simulink model "finaleproject_new_18"  (R2018b)
settings: Solver=VariableStepAuto  StartTime=0.0  StopTime=30  RelTol=1e-3
undefined symbols (not defined in the file): Ion, Lithium, sigbuilder_block
libraries: powerlib x21, simulink x6, electricdrivelib x2, powerlib_meascontrol x1, eePwmGenerator x1, re_lib x1
settings Model: Creator=ACER  LastModifiedBy=ACER
settings SolverCC: ZeroCrossAlgorithm=Adaptive
settings DataIOCC: ReturnWorkspaceOutputs=on
settings DebuggingCC: IgnoredZcDiagnostic=none  UnconnectedInputMsg=none  UnconnectedOutputMsg=none  UnconnectedLineMsg=none  SFMachineParentedDataDiag=error
settings ModelReferenceCC: EnableRefExpFcnMdlSchedulingChecks=off
settings RTWCC: Description=Generic Real-Time Target

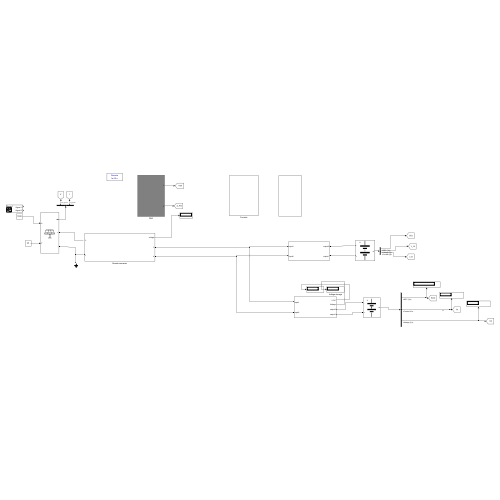
[thumbnail: Simulink's stored preview of the top-level diagram]
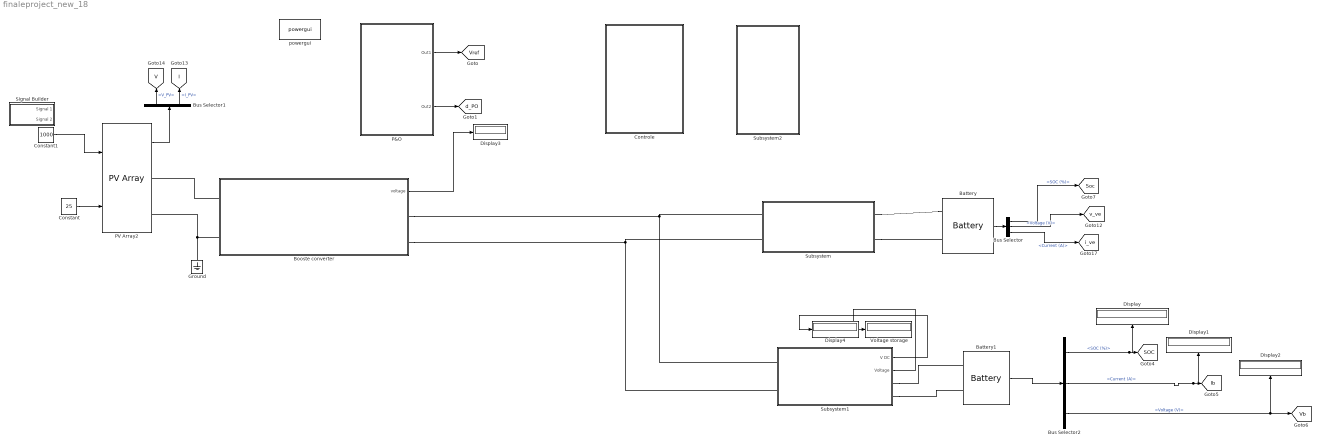
== system finaleproject_new_18 ==
  Battery : electricdrivelib/Extra Sources/Battery  BatType=Lithium-Ion  ShowTempParam=off  ThermalPreset=no  ShowAgeParam=off  NomV=400  NomQ=125  SOC=79.9  Batt_Tr=0.0001  PresetModel=on  MaxQ=125  MinV=300  FullV=465.5949  Dis_rate=54.3478  R=0.032  Normal_OP=113.0435  expZone="[432.1543      6.141304]"  current=[6.5 13 32.5]  Units=Time  Tci=20  NomT=20  T2=-30  MaxQ2=4.8  FullV2=7.1  Normal_OP2=5.655  expZone2="[6.58           1]"  Rca=0.6  ti=2000  Dp=0  Neq0=0  Tsim=1e6  Ta1=25  Qeol=5.4*0.9  Reol=0.013333*1.2  Char_age=[2.3478, 3]  Dis_age=[2.3478, 10]  N1=1500  N2=10500  N3=1000  N4=1400  Ta2=45  N5=950
  Battery1 : electricdrivelib/Extra Sources/Battery  BatType=Lithium-Ion  ShowTempParam=off  ThermalPreset=no  ShowAgeParam=off  NomV=300  NomQ=200*6  SOC=80  Batt_Tr=0.0001  PresetModel=on  MaxQ=1200  MinV=225  FullV=349.1961  Dis_rate=521.7391  R=0.0025  Normal_OP=1085.2174  expZone="[324.1158      58.95652]"  current=[6.5 13 32.5]  Units=Time  Tci=20  NomT=20  T2=-30  MaxQ2=4.8  FullV2=7.1  Normal_OP2=5.655  expZone2="[6.58           1]"  Rca=0.6  ti=2000  Dp=0  Neq0=0  Tsim=1e6  Ta1=25  Qeol=5.4*0.9  Reol=0.013333*1.2  Char_age=[2.3478, 3]  Dis_age=[2.3478, 10]  N1=1500  N2=10500  N3=1000  N4=1400  Ta2=45  N5=950
  Booste converter : Subsystem
  Bus Selector : BusSelector  OutputSignals=SOC (%),Voltage (V),Current (A)
  Bus Selector1 : BusSelector  OutputSignals=V_PV,I_PV
  Bus Selector2 : BusSelector  OutputSignals=SOC (%),Current (A),Voltage (V)
  Constant : Constant  Value=25
  Constant1 : Constant  Value=1000
  Controle : Subsystem
  Display{,1..4} (5 alike) : Display
  Ground : powerlib/Elements/Ground  LConnTagsString=a
  P&O : Subsystem
  PV Array2 : re_lib/Solar/PV Array  Npar=8*6  Nser=10  PlotType=array @ 1000 W/m2 & specified temperatures  S_vec="[ 1000  500  100 ]"  Temp_C_vec="[  25  ]"  ModuleName=User-defined  PlotWhenSelected=off  Pm=210.18  Ncell=72  Voc=45.90  Isc=6  Vm=37.20  Im=5.65  beta_Voc_pc=-0.36099  alpha_Isc_pc=0.102  beta_Voc=-0.16569  alpha_Isc=0.00612  IL=6.0381  I0=2.2435e-10  nI=1.0339  Rsh=465.1473  Rs=0.54298  RobustModel=off  RobustCellTemperature=25  BAL=on  Tc=1e-6  Tfilter=5e-5
  Signal Builder : Subsystem  Tag=STV Subsys  LoadFcn=sigbuilder_block('load');  StartFcn=sigbuilder_block('start');  StopFcn=sigbuilder_block('stop');  ClipboardFcn=sigbuilder_block('clipboard');  mask(Sigbuilder block){tuvar=[0:10]}
      mask help: Simulink:masks:SigbuilderBlock_MD
      mask init:
      | if ~strcmp(get_param(bdroot(gcbh),'SimulationStatus'),'stopped') tuvar = sigbuilder_block('maskInit'); end
      settings: CopyFcn=sigbuilder_block('copy');  DeleteFcn=sigbuilder_block('delete');  ModelCloseFcn=sigbuilder_block('modelClose');  PreSaveFcn=sigbuilder_block('preSave');  PauseFcn=sigbuilder_block('pause');  ContinueFcn=sigbuilder_block('continue');  NameChangeFcn=sigbuilder_block('namechange');  OpenFcn=sigbuilder_block('open',[204.5 106 550.5 362.5 ]);  CloseFcn=sigbuilder_block('close');
      mask Display: plot(0, 0, 100, 100,[2, 2, 32, 32, 2], [68, 8, 8, 68, 68],[32, 2], [38, 38], [32, 19, 2],[53, 60, 44], [32, 17, 17, 2],[16, 16, 31, 31]);txt = getActiveGroup(gcbh);text(2, 100, txt,'verticalAlignment', 'top');
  Subsystem : Subsystem
  Subsystem1 : Subsystem
  Subsystem2 : Subsystem
  Voltage storage : Display
  powergui : powerlib/powergui  Priority=1  SimulationMode=Discrete  SampleTime=10e-6  frequency=60  Iterations=50  frequencyindice=0  Pbase=100e6  ErrMax=1e-4  UnitsV=kV  UnitsW=MW  buscounter=0  FunctionMessages=off  echomessages=off  EnableUseOfTLC=off  CurrentSourceSwitches=off  DisableSnubberDevices=off  DisableRonSwitches=off  DisableVfSwitches=off  DisplayEquations=off  AutomaticDiscreteSolvers=off  SolverType=Tustin/Backward Euler (TBE)  Interpol=off  ExternalGateDelay=off  methode=off  Ts=100  x0status=blocks  SPID=on  SwTol=0  HookPort=off  NonlinearTolerance=1e-4  nMaxIteration=100  ContinueOnMaxIteration=off  RestoreLinks=warning  ResistiveCurrentMeasurement=off  Frange=[0:2:500]  Ylog=off  Xlog=on  ShowGrid=off  save=off  variable=ZData  structure=0  ZoomFFT=off  StartTime=0.0  cycles=1  DisplayStyle=1  fundamental=60  FreqAxis=off  MaxFrequency=1000  frequencyindicesteady=1  RmsSteady=1  display=off
  tag scope: I=global, Ib=global, SOC=global, Soc=global, V=global, Vb=global, Vref=global, d_PO=global, i_ve=global, v_ve=global
  wires:
  Constant1/1 -> PV Array2/1
  Bus Selector2/2 -> [Ib], Display1/1  "<Current (A)>"
  Bus Selector/2 -> [v_ve]  "<Voltage (V)>"
  Battery/1 -> Bus Selector/1
  P&O/2(Out2) -> [d_PO]
  PV Array2/1 -> Bus Selector1/1
  Bus Selector/1 -> [Soc]  "<SOC (%)>"
  Bus Selector/3 -> [i_ve]  "<Current (A)>"
  Bus Selector1/1 -> [V]  "<V_PV>"
  Bus Selector2/3 -> [Vb], Display2/1  "<Voltage (V)>"
  Constant/1 -> PV Array2/2
  Battery1/1 -> Bus Selector2/1
  Booste converter/1(voltage) -> Display3/1
  Bus Selector1/2 -> [I]  "<I_PV>"
  P&O/1(Out1) -> [Vref]
  Bus Selector2/1 -> Display/1, [SOC]  "<SOC (%)>"
  Subsystem1/2(Voltage) -> Voltage storage/1
  Subsystem1/1(V DC) -> Display4/1
  connections:
  Booste converter/LConn2 -- PV Array2/RConn2 -- Ground/LConn1
  Subsystem/RConn1 -- Battery/LConn2
  Subsystem/RConn2 -- Battery/LConn1
  Subsystem1/RConn1 -- Battery1/LConn2
  Booste converter/LConn1 -- PV Array2/RConn1
  Subsystem1/RConn2 -- Battery1/LConn1
  Booste converter/RConn1 -- Subsystem/LConn1 -- Subsystem1/LConn1
  Booste converter/RConn2 -- Subsystem/LConn2 -- Subsystem1/LConn2

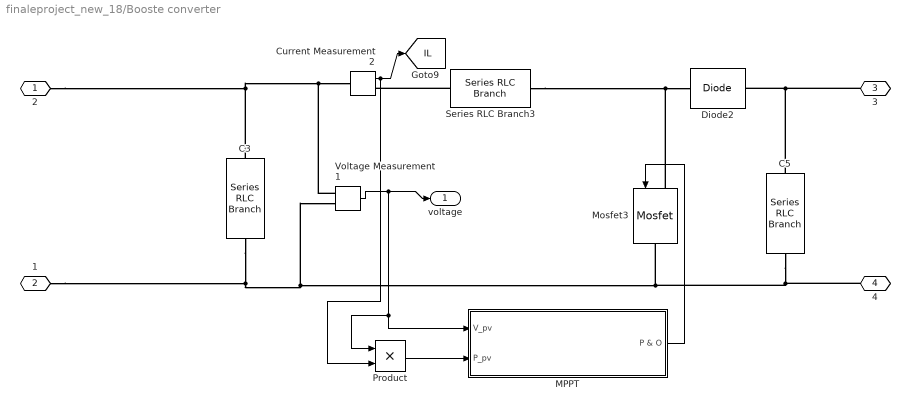
== system finaleproject_new_18/Booste converter ==
  C3 : powerlib/Elements/Series RLC Branch  LConnTagsString=__new0  RConnTagsString=__new0  BranchType=C  Resistance=0.1  Inductance=0.0078  SetiL0=off  InitialCurrent=0  Capacitance=470e-6  Setx0=on  InitialVoltage=400  Measurements=None
  C5 : powerlib/Elements/Series RLC Branch  LConnTagsString=__new0  RConnTagsString=__new0  BranchType=C  Resistance=0.1  Inductance=0.0078  SetiL0=off  InitialCurrent=0  Capacitance=222e-6  Setx0=off  InitialVoltage=500  Measurements=None
  Current Measurement2 : powerlib/Measurements/Current Measurement  PhasorSimulation=off  OutputType=Complex  PSBequivalent=0
  Diode2 : powerlib/Power Electronics/Diode  Ron=0.001  Lon=0  Vf=0.8  IC=0  UseSnubber=off  Rs=500  Cs=250e-9  Measurements=off
  MPPT : Subsystem
  Mosfet3 : powerlib/Power Electronics/Mosfet  Ron=0.1  Lon=0  Rd=0.01  Vfd=0  IC=0  Rs=1e5  Cs=inf  Measurements=off
  Product : Product
  Series RLC Branch3 : powerlib/Elements/Series RLC Branch  LConnTagsString=__new0  RConnTagsString=__new0  BranchType=L  Resistance=0.1  Inductance=2.25e-3  SetiL0=off  InitialCurrent=0  Capacitance=1e-6  Setx0=off  InitialVoltage=0  Measurements=None
  Voltage Measurement1 : powerlib/Measurements/Voltage Measurement  PhasorSimulation=off  OutputType=Complex  PSBequivalent=0
  2 : PMIOPort  Side=Left
  1 : PMIOPort  Port=2  Side=Left
  3 : PMIOPort  Port=3  Side=Right
  4 : PMIOPort  Port=4  Side=Right
  voltage : Outport
  tag scope: IL=global
  wires:
  Current Measurement2/1 -> Product/2, [IL]
  Voltage Measurement1/1 -> Product/1, MPPT/1(V_pv), voltage/1
  Product/1 -> MPPT/2(P_pv)
  MPPT/1(P & O) -> Mosfet3/1
  connections:
  Series RLC Branch3/RConn1 -- Diode2/LConn1 -- Mosfet3/LConn1
  C5/LConn1 -- Diode2/RConn1 -- 3/RConn1
  Voltage Measurement1/LConn1 -- C3/LConn1 -- 2/RConn1 -- Current Measurement2/LConn1
  4/RConn1 -- C5/RConn1 -- Mosfet3/RConn1 -- C3/RConn1 -- 1/RConn1 -- Voltage Measurement1/LConn2
  Series RLC Branch3/LConn1 -- Current Measurement2/RConn1

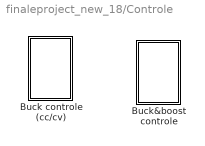
== system finaleproject_new_18/Controle ==
  "Buck controle (cc/cv) " : Subsystem
  Buck&boost controle : Subsystem

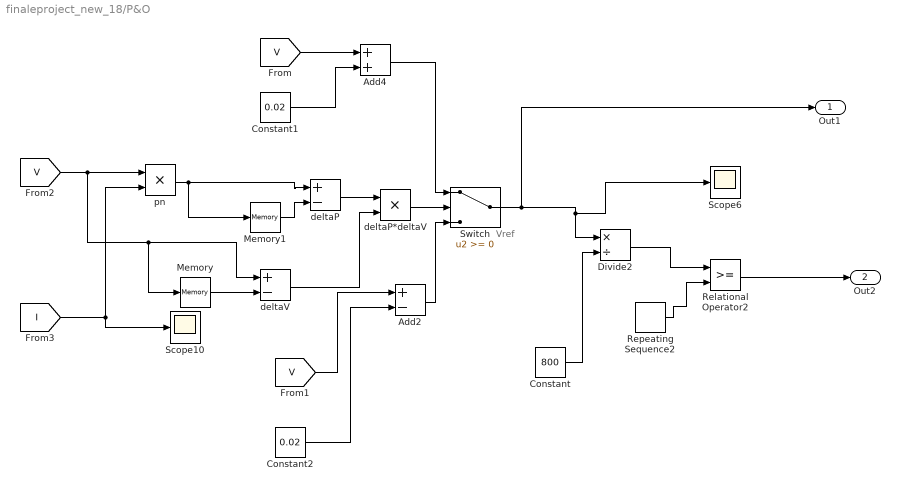
== system finaleproject_new_18/P&O ==
  note: Vref
  Add2 : Sum  Inputs=+-
  Add4 : Sum
  Constant : Constant  Value=800
  Constant1 : Constant  Value=0.02
  Constant2 : Constant  Value=0.02
  Divide2 : Product  Inputs=*/
  Memory : Memory
  Memory1 : Memory
  Relational Operator2 : RelationalOperator  OutDataTypeStr=boolean  RndMeth=Nearest
  Repeating Sequence2 : simulink/Sources/Repeating Sequence  rep_seq_t=[0 1/5000]  rep_seq_y=[0 1]
  Scope10 : Scope
  Scope6 : Scope
  Switch : Switch
  deltaP : Sum  Inputs=+-
  deltaP*deltaV : Product
  deltaV : Sum  Inputs=+-
  pn : Product
  Out1 : Outport  VectorParamsAs1DForOutWhenUnconnected=off
  Out2 : Outport  Port=2  VectorParamsAs1DForOutWhenUnconnected=off
  wires:
  pn/1 -> Memory1/1, deltaP/1
  Constant1/1 -> Add4/2
  Add2/1 -> Switch/3
  deltaP*deltaV/1 -> Switch/2
  [V] -> Add4/1
  Add4/1 -> Switch/1
  deltaP/1 -> deltaP*deltaV/1
  [V] -> deltaV/1, Memory/1, pn/1
  [I] -> pn/2, Scope10/1
  deltaV/1 -> deltaP*deltaV/2
  Memory/1 -> deltaV/2
  Relational Operator2/1 -> Out2/1
  Constant2/1 -> Add2/2
  [V] -> Add2/1
  Repeating Sequence2/1 -> Relational Operator2/2
  Divide2/1 -> Relational Operator2/1
  Memory1/1 -> deltaP/2
  Switch/1 -> Out1/1, Scope6/1, Divide2/1
  Constant/1 -> Divide2/2

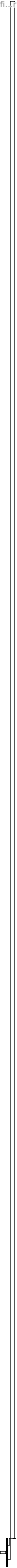
== system finaleproject_new_18/Signal Builder ==
  Demux : Demux  Tag=STV Demux  Outputs=2
      settings: DisplayOption=none
  FromWs : FromWorkspace  Tag=STV FromWs  VariableName=tuvar
      SigBuilderData=|
      | common.afterFinalStr = 'Extrapolate'
      | common.sampleTime = 0
      | dataSet.timeRange = [0 30]
      | dataSet.name = 'Group 1'
      | sbobj.Groups.Name = 'Group 1'
      | sbobj.Groups.Signals(1).Name = 'Signal 1'
      | sbobj.Groups.Signals(1).XData = [0 4 9.85 11 12 12 30]
      | sbobj.Groups.Signals(1).YData = [1000 1005 925 865 760 195 205]
      | sbobj.Groups.Signals(2).Name = 'Signal 2'
      | sbobj.Groups.Signals(2).XData = [0 5 5 30]
      | sbobj.Groups.Signals(2).YData = [0 0 1 1]
      | sbobj.Groups.TimeRange = [0 30]
  Signal 1 : Outport  Tag=STV Outport
  Signal 2 : Outport  Tag=STV Outport  Port=2
  wires:
  Demux/1 -> Signal 1/1
  FromWs/1 -> Demux/1
  Demux/2 -> Signal 2/1

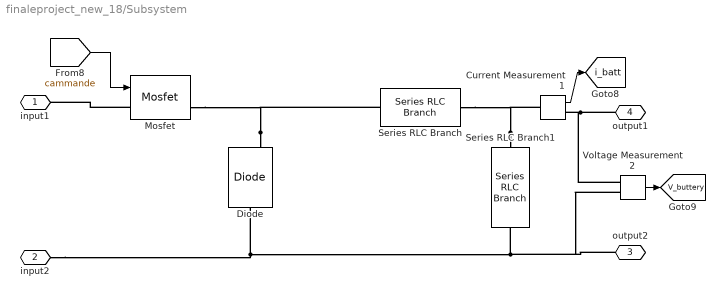
== system finaleproject_new_18/Subsystem ==
  Current Measurement1 : powerlib/Measurements/Current Measurement  PhasorSimulation=off  OutputType=Complex  PSBequivalent=0
  Diode : powerlib/Power Electronics/Diode  Ron=0.001  Lon=0  Vf=0.8  IC=0  UseSnubber=0  Rs=500  Cs=250e-9  Measurements=on
  Mosfet : powerlib/Power Electronics/Mosfet  Ron=0.1  Lon=0  Rd=0.01  Vfd=0  IC=0  Rs=1e5  Cs=inf  Measurements=on
  Series RLC Branch : powerlib/Elements/Series RLC Branch  LConnTagsString=__new0  RConnTagsString=__new0  BranchType=L  Resistance=1  Inductance=2.13e-3  SetiL0=off  InitialCurrent=0  Capacitance=1e-6  Setx0=off  InitialVoltage=0  Measurements=None
  Series RLC Branch1 : powerlib/Elements/Series RLC Branch  LConnTagsString=__new0  RConnTagsString=__new0  BranchType=C  Resistance=1  Inductance=1e-3  SetiL0=off  InitialCurrent=0  Capacitance=47e-6  Setx0=off  InitialVoltage=0  Measurements=None
  Voltage Measurement2 : powerlib/Measurements/Voltage Measurement  PhasorSimulation=off  OutputType=Complex  PSBequivalent=0
  input1 : PMIOPort  Side=Left
  input2 : PMIOPort  Port=2  Side=Left
  output2 : PMIOPort  Port=3  Side=Right
  output1 : PMIOPort  Port=4  Side=Right
  tag scope: V_buttery=global, i_batt=global
  wires:
  Current Measurement1/1 -> [i_batt]
  [cammande] -> Mosfet/1
  Voltage Measurement2/1 -> [V_buttery]
  connections:
  Voltage Measurement2/LConn1 -- output1/RConn1 -- Current Measurement1/RConn1
  Series RLC Branch1/LConn1 -- Series RLC Branch/RConn1 -- Current Measurement1/LConn1
  Diode/RConn1 -- Mosfet/RConn1 -- Series RLC Branch/LConn1
  input2/RConn1 -- Diode/LConn1 -- Voltage Measurement2/LConn2 -- output2/RConn1 -- Series RLC Branch1/RConn1
  Mosfet/LConn1 -- input1/RConn1

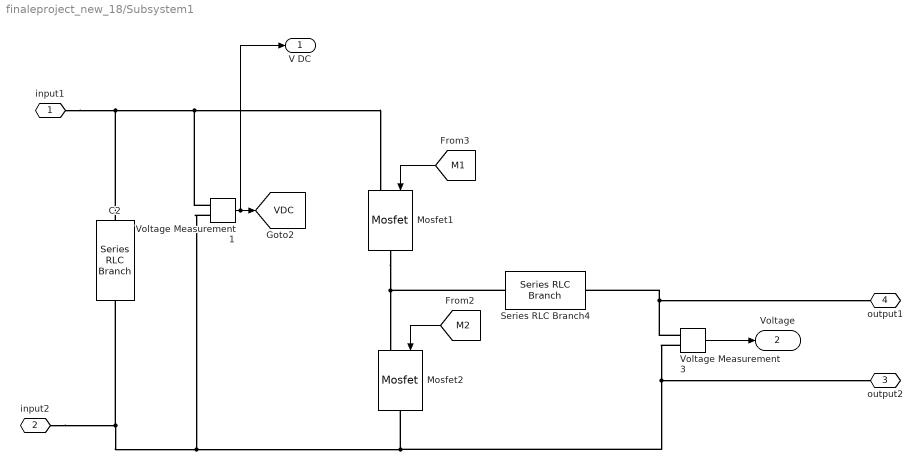
== system finaleproject_new_18/Subsystem1 ==
  C2 : powerlib/Elements/Series RLC Branch  LConnTagsString=__new0  RConnTagsString=__new0  BranchType=C  Resistance=0.01  Inductance=0.0078  SetiL0=off  InitialCurrent=0  Capacitance=5000e-6  Setx0=off  InitialVoltage=0  Measurements=None
  Mosfet1 : powerlib/Power Electronics/Mosfet  Ron=0.1  Lon=0  Rd=0.01  Vfd=0  IC=0  Rs=1e5  Cs=inf  Measurements=off
  Mosfet2 : powerlib/Power Electronics/Mosfet  Ron=0.1  Lon=0  Rd=0.01  Vfd=0  IC=0  Rs=1e5  Cs=inf  Measurements=off
  Series RLC Branch4 : powerlib/Elements/Series RLC Branch  LConnTagsString=__new0  RConnTagsString=__new0  BranchType=L  Resistance=0.05  Inductance=2.2e-3  SetiL0=off  InitialCurrent=0  Capacitance=1e-6  Setx0=off  InitialVoltage=0  Measurements=None
  Voltage Measurement1 : powerlib/Measurements/Voltage Measurement  PhasorSimulation=off  OutputType=Complex  PSBequivalent=0
  Voltage Measurement3 : powerlib/Measurements/Voltage Measurement  PhasorSimulation=off  OutputType=Complex  PSBequivalent=0
  input1 : PMIOPort  Side=Left
  input2 : PMIOPort  Port=2  Side=Left
  output2 : PMIOPort  Port=3  Side=Right
  output1 : PMIOPort  Port=4  Side=Right
  V DC : Outport
  Voltage : Outport  Port=2
  tag scope: VDC=global
  wires:
  Voltage Measurement3/1 -> Voltage/1
  [M1] -> Mosfet1/1
  [M2] -> Mosfet2/1
  Voltage Measurement1/1 -> V DC/1, [VDC]
  connections:
  input2/RConn1 -- Voltage Measurement1/LConn2 -- Voltage Measurement3/LConn2 -- output2/RConn1 -- Mosfet2/RConn1 -- C2/RConn1
  Series RLC Branch4/LConn1 -- Mosfet1/RConn1 -- Mosfet2/LConn1
  C2/LConn1 -- input1/RConn1 -- Voltage Measurement1/LConn1 -- Mosfet1/LConn1
  Voltage Measurement3/LConn1 -- output1/RConn1 -- Series RLC Branch4/RConn1

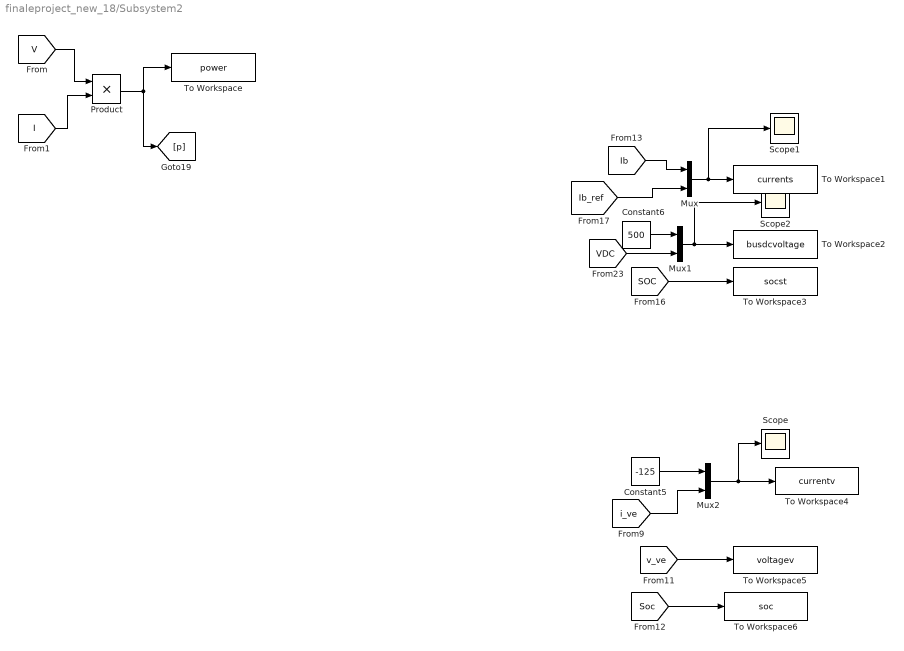
== system finaleproject_new_18/Subsystem2 ==
  Constant5 : Constant  Value=-125
  Constant6 : Constant  Value=500
  Mux : Mux  Inputs=2
  Mux1 : Mux  Inputs=2
  Mux2 : Mux  Inputs=2
  Product : Product
  Scope : Scope
  Scope1 : Scope
  Scope2 : Scope
  To Workspace : ToWorkspace  VariableName=power  SaveFormat=Timeseries  SampleTime=-1
  To Workspace1 : ToWorkspace  VariableName=currents  SaveFormat=Timeseries  SampleTime=-1
  To Workspace2 : ToWorkspace  VariableName=busdcvoltage  SaveFormat=Timeseries  SampleTime=-1
  To Workspace3 : ToWorkspace  VariableName=socst  SaveFormat=Timeseries  SampleTime=-1
  To Workspace4 : ToWorkspace  VariableName=currentv  SaveFormat=Timeseries  SampleTime=-1
  To Workspace5 : ToWorkspace  VariableName=voltagev  SaveFormat=Timeseries  SampleTime=-1
  To Workspace6 : ToWorkspace  VariableName=soc  SaveFormat=Timeseries  SampleTime=-1
  wires:
  [Ib] -> Mux/1
  Constant6/1 -> Mux1/1
  [Ib_ref] -> Mux/2
  [VDC] -> Mux1/2
  [i_ve] -> Mux2/2
  Constant5/1 -> Mux2/1
  [V] -> Product/1
  Product/1 -> To Workspace/1, [p]
  [I] -> Product/2
  Mux/1 -> Scope1/1, To Workspace1/1
  [SOC] -> To Workspace3/1
  Mux1/1 -> Scope2/1, To Workspace2/1
  Mux2/1 -> Scope/1, To Workspace4/1
  [v_ve] -> To Workspace5/1
  [Soc] -> To Workspace6/1

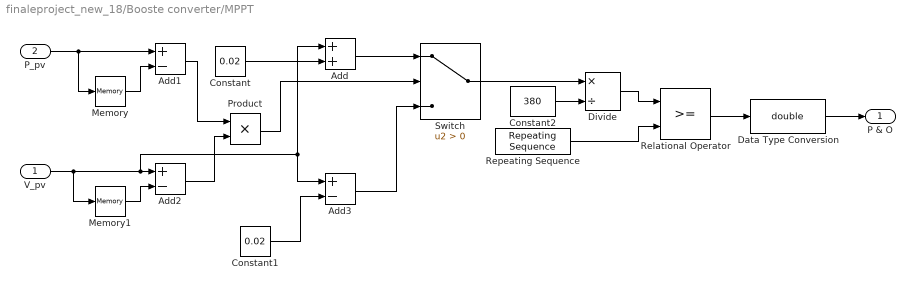
== system finaleproject_new_18/Booste converter/MPPT ==
  V_pv : Inport
  P_pv : Inport  Port=2
  Add : Sum
  Add1 : Sum  Inputs=+-
  Add2 : Sum  Inputs=+-
  Add3 : Sum  Inputs=+-
  Constant : Constant  Value=0.02
  Constant1 : Constant  Value=0.02
  Constant2 : Constant  Value=380
  Data Type Conversion : DataTypeConversion  OutDataTypeStr=double
  Divide : Product  Inputs=*/
  Memory : Memory
  Memory1 : Memory
  Product : Product
  Relational Operator : RelationalOperator  OutDataTypeStr=boolean  RndMeth=Nearest
  Repeating Sequence : simulink/Sources/Repeating Sequence  rep_seq_t=[0 1/5000]  rep_seq_y=[0 1]
  Switch : Switch  Criteria=u2 > Threshold
  P & O : Outport  VectorParamsAs1DForOutWhenUnconnected=off
  wires:
  Switch/1 -> Divide/1
  Add/1 -> Switch/1
  Divide/1 -> Relational Operator/1
  Constant2/1 -> Divide/2
  Data Type Conversion/1 -> P & O/1
  Add2/1 -> Product/2
  Constant/1 -> Add/2
  Add3/1 -> Switch/3
  Add1/1 -> Product/1
  P_pv/1 -> Add1/1, Memory/1
  Product/1 -> Switch/2
  Relational Operator/1 -> Data Type Conversion/1
  Constant1/1 -> Add3/2
  Memory1/1 -> Add2/2
  Memory/1 -> Add1/2
  Repeating Sequence/1 -> Relational Operator/2
  V_pv/1 -> Add3/1, Add/1, Add2/1, Memory1/1

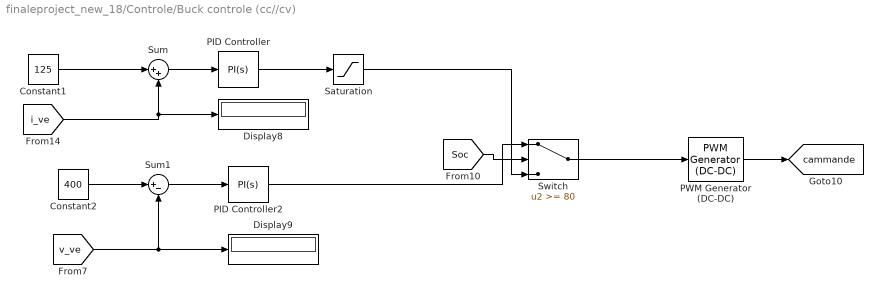
== system finaleproject_new_18/Controle/Buck controle (cc//cv)  ==
  Constant1 : Constant  Value=125
  Constant2 : Constant  Value=400
  Display8 : Display
  Display9 : Display
  PID Controller : simulink/Continuous/PID Controller  Controller=PI  Form=Parallel  TimeDomain=Continuous-time  SampleTime=-1  IntegratorMethod=Forward Euler  ControllerParametersSource=internal  P=7  I=5000  D=0  N=100  UseFilter=on  TunerSelectOption=Transfer Function Based (PID Tuner App)  InitialConditionSource=internal  InitialConditionForIntegrator=0  InitialConditionForFilter=0  DifferentiatorICPrevScaledInput=0  ExternalReset=none  TrackingMode=off  Kt=1  LimitOutput=off  UpperSaturationLimit=inf  LowerSaturationLimit=-inf  LinearizeAsGain=on  AntiWindupMode=none  Kb=1  POutMin=[]  POutMax=[]  IOutMin=[]  IOutMax=[]  DOutMin=[]  DOutMax=[]  NOutMin=[]  NOutMax=[]  SumOutMin=[]  SumOutMax=[]  SaturationOutMin=[]  SaturationOutMax=[]  PParamMin=[]  PParamMax=[]  IParamMin=[]  IParamMax=[]  DParamMin=[]  DParamMax=[]  NParamMin=[]  NParamMax=[]  KbParamMin=[]  KbParamMax=[]  KtParamMin=[]  KtParamMax=[]  KbOutMin=[]  KbOutMax=[]  KtOutMin=[]  KtOutMax=[]  IntegratorOutMin=[]  IntegratorOutMax=[]  FilterOutMin=[]  FilterOutMax=[]  SumI1OutMin=[]  SumI1OutMax=[]  SumI2OutMin=[]  SumI2OutMax=[]  SumI3OutMin=[]  SumI3OutMax=[]  SumI4OutMin=[]  SumI4OutMax=[]  SumDOutMin=[]  SumDOutMax=[]  DifferentiatorOutMin=[]  DifferentiatorOutMax=[]  FilterDiffOutCoefMin=[]  FilterDiffOutCoefMax=[]  ReciprocalOutMin=[]  ReciprocalOutMax=[]  SumDenOutMin=[]  SumDenOutMax=[]  SumNumOutMin=[]  SumNumOutMax=[]  DivideOutMin=[]  DivideOutMax=[]  IntegratorContinuousStateAttributes=''  IntegratorStateMustResolveToSignalObject=off  IntegratorRTWStateStorageClass=Auto  FilterContinuousStateAttributes=''  FilterStateMustResolveToSignalObject=off  FilterRTWStateStorageClass=Auto  ParallelPVariant=InternalParameters  IdealPVariant=Disabled  IVariant=InternalParameters  DVariant=Disabled  IntegratorVariant=Continuous  SatVariant=Disabled  AWVariant=Passthrough  PCopyVariant=Disabled  TRVariant=Disabled  FdbkBlocksVariant=Forward  IdealPFdbkVariant=Disabled  SatFdbkVariant=Disabled  DerivativeFilterVariant=Disabled  NVariant=Disabled  NCopyVariant=Disabled_SignalSpec  FilterICVariant=Disabled  IntegratorICVariant=InternalICs  ExternalResetVariant=Disabled  TRSumVariant=Passthrough  SumFdbkVariant=Disabled  SumVariant=Sum_PI
  PID Controller2 : simulink/Continuous/PID Controller  Controller=PI  Form=Parallel  TimeDomain=Continuous-time  SampleTime=-1  IntegratorMethod=Forward Euler  ControllerParametersSource=internal  P=1.1  I=210  D=0  N=100  UseFilter=on  TunerSelectOption=Transfer Function Based (PID Tuner App)  InitialConditionSource=internal  InitialConditionForIntegrator=0  InitialConditionForFilter=0  DifferentiatorICPrevScaledInput=0  ExternalReset=none  TrackingMode=off  Kt=1  LimitOutput=off  UpperSaturationLimit=inf  LowerSaturationLimit=-inf  LinearizeAsGain=on  AntiWindupMode=none  Kb=1  POutMin=[]  POutMax=[]  IOutMin=[]  IOutMax=[]  DOutMin=[]  DOutMax=[]  NOutMin=[]  NOutMax=[]  SumOutMin=[]  SumOutMax=[]  SaturationOutMin=[]  SaturationOutMax=[]  PParamMin=[]  PParamMax=[]  IParamMin=[]  IParamMax=[]  DParamMin=[]  DParamMax=[]  NParamMin=[]  NParamMax=[]  KbParamMin=[]  KbParamMax=[]  KtParamMin=[]  KtParamMax=[]  KbOutMin=[]  KbOutMax=[]  KtOutMin=[]  KtOutMax=[]  IntegratorOutMin=[]  IntegratorOutMax=[]  FilterOutMin=[]  FilterOutMax=[]  SumI1OutMin=[]  SumI1OutMax=[]  SumI2OutMin=[]  SumI2OutMax=[]  SumI3OutMin=[]  SumI3OutMax=[]  SumI4OutMin=[]  SumI4OutMax=[]  SumDOutMin=[]  SumDOutMax=[]  DifferentiatorOutMin=[]  DifferentiatorOutMax=[]  FilterDiffOutCoefMin=[]  FilterDiffOutCoefMax=[]  ReciprocalOutMin=[]  ReciprocalOutMax=[]  SumDenOutMin=[]  SumDenOutMax=[]  SumNumOutMin=[]  SumNumOutMax=[]  DivideOutMin=[]  DivideOutMax=[]  IntegratorContinuousStateAttributes=''  IntegratorStateMustResolveToSignalObject=off  IntegratorRTWStateStorageClass=Auto  FilterContinuousStateAttributes=''  FilterStateMustResolveToSignalObject=off  FilterRTWStateStorageClass=Auto  ParallelPVariant=InternalParameters  IdealPVariant=Disabled  IVariant=InternalParameters  DVariant=Disabled  IntegratorVariant=Continuous  SatVariant=Disabled  AWVariant=Passthrough  PCopyVariant=Disabled  TRVariant=Disabled  FdbkBlocksVariant=Forward  IdealPFdbkVariant=Disabled  SatFdbkVariant=Disabled  DerivativeFilterVariant=Disabled  NVariant=Disabled  NCopyVariant=Disabled_SignalSpec  FilterICVariant=Disabled  IntegratorICVariant=InternalICs  ExternalResetVariant=Disabled  TRSumVariant=Passthrough  SumFdbkVariant=Disabled  SumVariant=Sum_PI
  PWM Generator (DC-DC) : powerlib_meascontrol/Pulse & Signal Generators/PWM Generator (DC-DC)  Fsw=5000  Ts=0
  Saturation : Saturate  UpperLimit=0.95  LowerLimit=0.05
  Sum : Sum  Inputs=|++
  Sum1 : Sum  Inputs=|+-
  Switch : Switch  Threshold=80
  tag scope: cammande=global
  wires:
  Sum1/1 -> PID Controller2/1
  Constant2/1 -> Sum1/1
  Saturation/1 -> Switch/3
  PWM Generator (DC-DC)/1 -> [cammande]
  PID Controller/1 -> Saturation/1
  Sum/1 -> PID Controller/1
  [v_ve] -> Display9/1, Sum1/2
  [i_ve] -> Display8/1, Sum/2
  [Soc] -> Switch/2
  Switch/1 -> PWM Generator (DC-DC)/1
  PID Controller2/1 -> Switch/1
  Constant1/1 -> Sum/1

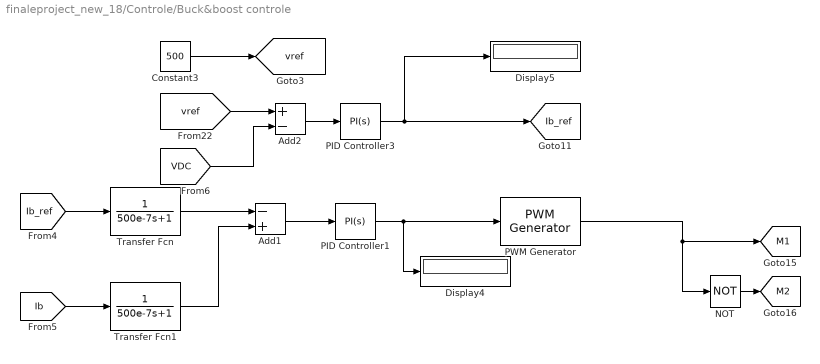
== system finaleproject_new_18/Controle/Buck&boost controle ==
  Add1 : Sum  Inputs=-+
  Add2 : Sum  Inputs=+-
  Constant3 : Constant  Value=500
  Display4 : Display
  Display5 : Display
  NOT : Logic  Operator=NOT  IconShape=distinctive  AllPortsSameDT=off  OutDataTypeStr=boolean
  PID Controller1 : simulink/Continuous/PID Controller  Controller=PI  Form=Parallel  TimeDomain=Continuous-time  SampleTime=-1  IntegratorMethod=Forward Euler  ControllerParametersSource=internal  P=0.03  I=250  D=0  N=100  UseFilter=on  TunerSelectOption=Frequency Response Based  InitialConditionSource=internal  InitialConditionForIntegrator=0  InitialConditionForFilter=0  DifferentiatorICPrevScaledInput=0  ExternalReset=none  TrackingMode=off  Kt=1  LimitOutput=on  UpperSaturationLimit=0.95  LowerSaturationLimit=0  LinearizeAsGain=on  AntiWindupMode=clamping  Kb=1  POutMin=[]  POutMax=[]  IOutMin=[]  IOutMax=[]  DOutMin=[]  DOutMax=[]  NOutMin=[]  NOutMax=[]  SumOutMin=[]  SumOutMax=[]  SaturationOutMin=[]  SaturationOutMax=[]  PParamMin=[]  PParamMax=[]  IParamMin=[]  IParamMax=[]  DParamMin=[]  DParamMax=[]  NParamMin=[]  NParamMax=[]  KbParamMin=[]  KbParamMax=[]  KtParamMin=[]  KtParamMax=[]  KbOutMin=[]  KbOutMax=[]  KtOutMin=[]  KtOutMax=[]  IntegratorOutMin=[]  IntegratorOutMax=[]  FilterOutMin=[]  FilterOutMax=[]  SumI1OutMin=[]  SumI1OutMax=[]  SumI2OutMin=[]  SumI2OutMax=[]  SumI3OutMin=[]  SumI3OutMax=[]  SumI4OutMin=[]  SumI4OutMax=[]  SumDOutMin=[]  SumDOutMax=[]  DifferentiatorOutMin=[]  DifferentiatorOutMax=[]  FilterDiffOutCoefMin=[]  FilterDiffOutCoefMax=[]  ReciprocalOutMin=[]  ReciprocalOutMax=[]  SumDenOutMin=[]  SumDenOutMax=[]  SumNumOutMin=[]  SumNumOutMax=[]  DivideOutMin=[]  DivideOutMax=[]  IntegratorContinuousStateAttributes=''  IntegratorStateMustResolveToSignalObject=off  IntegratorRTWStateStorageClass=Auto  FilterContinuousStateAttributes=''  FilterStateMustResolveToSignalObject=off  FilterRTWStateStorageClass=Auto  ParallelPVariant=InternalParameters  IdealPVariant=Disabled  IVariant=InternalParameters  DVariant=Disabled  IntegratorVariant=Continuous  SatVariant=Enabled  AWVariant=ContClampingParallel  PCopyVariant=Disabled  TRVariant=Disabled  FdbkBlocksVariant=Forward  IdealPFdbkVariant=Disabled  SatFdbkVariant=Disabled  DerivativeFilterVariant=Disabled  NVariant=Disabled  NCopyVariant=Disabled_SignalSpec  FilterICVariant=Disabled  IntegratorICVariant=InternalICs  ExternalResetVariant=Disabled  TRSumVariant=Passthrough  SumFdbkVariant=Disabled  SumVariant=Sum_PI
  PID Controller3 : simulink/Continuous/PID Controller  Controller=PI  Form=Parallel  TimeDomain=Continuous-time  SampleTime=-1  IntegratorMethod=Forward Euler  ControllerParametersSource=internal  P=0.03  I=350  D=0  N=100  UseFilter=on  TunerSelectOption=Frequency Response Based  InitialConditionSource=internal  InitialConditionForIntegrator=0  InitialConditionForFilter=0  DifferentiatorICPrevScaledInput=0  ExternalReset=none  TrackingMode=off  Kt=1  LimitOutput=off  UpperSaturationLimit=100  LowerSaturationLimit=-100  LinearizeAsGain=on  AntiWindupMode=none  Kb=1  POutMin=[]  POutMax=[]  IOutMin=[]  IOutMax=[]  DOutMin=[]  DOutMax=[]  NOutMin=[]  NOutMax=[]  SumOutMin=[]  SumOutMax=[]  SaturationOutMin=[]  SaturationOutMax=[]  PParamMin=[]  PParamMax=[]  IParamMin=[]  IParamMax=[]  DParamMin=[]  DParamMax=[]  NParamMin=[]  NParamMax=[]  KbParamMin=[]  KbParamMax=[]  KtParamMin=[]  KtParamMax=[]  KbOutMin=[]  KbOutMax=[]  KtOutMin=[]  KtOutMax=[]  IntegratorOutMin=[]  IntegratorOutMax=[]  FilterOutMin=[]  FilterOutMax=[]  SumI1OutMin=[]  SumI1OutMax=[]  SumI2OutMin=[]  SumI2OutMax=[]  SumI3OutMin=[]  SumI3OutMax=[]  SumI4OutMin=[]  SumI4OutMax=[]  SumDOutMin=[]  SumDOutMax=[]  DifferentiatorOutMin=[]  DifferentiatorOutMax=[]  FilterDiffOutCoefMin=[]  FilterDiffOutCoefMax=[]  ReciprocalOutMin=[]  ReciprocalOutMax=[]  SumDenOutMin=[]  SumDenOutMax=[]  SumNumOutMin=[]  SumNumOutMax=[]  DivideOutMin=[]  DivideOutMax=[]  IntegratorContinuousStateAttributes=''  IntegratorStateMustResolveToSignalObject=off  IntegratorRTWStateStorageClass=Auto  FilterContinuousStateAttributes=''  FilterStateMustResolveToSignalObject=off  FilterRTWStateStorageClass=Auto  ParallelPVariant=InternalParameters  IdealPVariant=Disabled  IVariant=InternalParameters  DVariant=Disabled  IntegratorVariant=Continuous  SatVariant=Disabled  AWVariant=Passthrough  PCopyVariant=Disabled  TRVariant=Disabled  FdbkBlocksVariant=Forward  IdealPFdbkVariant=Disabled  SatFdbkVariant=Disabled  DerivativeFilterVariant=Disabled  NVariant=Disabled  NCopyVariant=Disabled_SignalSpec  FilterICVariant=Disabled  IntegratorICVariant=InternalICs  ExternalResetVariant=Disabled  TRSumVariant=Passthrough  SumFdbkVariant=Disabled  SumVariant=Sum_PI
  PWM Generator : eePwmGenerator/PWM Generator  CarrCount=Up  Tper=1/5000  Tdelay=0  Ts=0
  Transfer Fcn : TransferFcn  Denominator=[500e-7 1]
  Transfer Fcn1 : TransferFcn  Denominator=[500e-7 1]
  tag scope: Ib_ref=global, M1=global, M2=global, vref=global
  wires:
  Add1/1 -> PID Controller1/1
  Add2/1 -> PID Controller3/1
  [vref] -> Add2/1
  [Ib_ref] -> Transfer Fcn/1
  PWM Generator/1 -> NOT/1, [M1]
  NOT/1 -> [M2]
  [VDC] -> Add2/2
  PID Controller1/1 -> Display4/1, PWM Generator/1
  PID Controller3/1 -> Display5/1, [Ib_ref]
  Constant3/1 -> [vref]
  Transfer Fcn/1 -> Add1/1
  Transfer Fcn1/1 -> Add1/2
  [Ib] -> Transfer Fcn1/1
